simulink model "lab08"  (Simulink 5.0)
settings: Solver=ode45  StartTime=0.0  StopTime=50  RelTol=1e-3
libraries: simulink x1
settings Model: LastModifiedBy=Frank Gloria  RTWOptions="-aEnforceIntegerDowncast=1 -aExtMode=0 -aExtModeTesting=0 -aFoldNonRolledExpr=1 -aForceParamTrailComments=0 -aGenerateComments=1 -aGenerateReport=0 -aIgnoreCustomStorageClasses=1 -aIncDataTypeInIds=0 -aIncHierarchyInIds=0 -aInlineInvariantSignals=0 -aInlinedPrmAccess=\"Literals\" -aLocalBlockOutputs=1 -aLogVarNameModifier=\"rt_\" -aMaxRTWIdLen=31 -aPrefixModelToSubsysFcnNames=1 -aRTWVerbose=1 -aRollThreshold=5 -aShowEliminatedStatements=0"

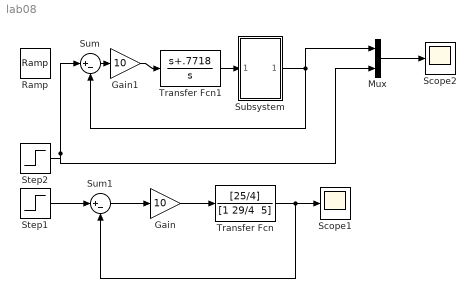
== system lab08 ==
  Gain : Gain  Gain=10  SaturateOnIntegerOverflow=on
  Gain1 : Gain  Gain=10  SaturateOnIntegerOverflow=on
  Mux : Mux  Inputs=2
  Ramp : simulink/Sources/Ramp  slope=1  start=0  X0=0
  Scope1 : Scope
  Scope2 : Scope
  Step1 : Step  Time=0  Before=1  SampleTime=0
  Step2 : Step  Time=0  Before=1  SampleTime=0
  Subsystem : Subsystem  mask{K=1/4}
      mask prompts: K "Ganho"
  Sum : Sum  Inputs=|+-  SaturateOnIntegerOverflow=on
  Sum1 : Sum  Inputs=|+-  SaturateOnIntegerOverflow=on
  Transfer Fcn : TransferFcn  Numerator=[25/4]  Denominator="[1 29/4  5]"
  Transfer Fcn1 : TransferFcn  Numerator=[1 .7718]  Denominator=[1 0]
  wires:
  Step1/1 -> Sum1/1
  Sum1/1 -> Gain/1
  Gain/1 -> Transfer Fcn/1
  Transfer Fcn1/1 -> Subsystem/1(In1)
  Subsystem/1(Out1) -> Sum/2, Mux/1
  Transfer Fcn/1 -> Scope1/1, Sum1/2
  Mux/1 -> Scope2/1
  Gain1/1 -> Transfer Fcn1/1
  Sum/1 -> Gain1/1
  Step2/1 -> Sum/1, Mux/2

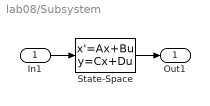
== system lab08/Subsystem ==
  In1 : Inport
  State-Space : StateSpace  A=[-7.5 5+7.5*K; -1 K]  B=[-5; 0]  C=[0 1+K]  D=0
  Out1 : Outport
  wires:
  In1/1 -> State-Space/1
  State-Space/1 -> Out1/1
